simulink model "part_d_sim"  (R2019a)
settings: Solver=FixedStepAuto  StartTime=0.0  StopTime=10.0  FixedStep=0.01  RelTol=1e-3
undefined symbols (not defined in the file): A, B, C, D, R, sigbuilder_block
settings Model: Creator=Ranjani Kripashankar  LastModifiedBy=reema
settings DataIOCC: ReturnWorkspaceOutputs=off
settings DebuggingCC: ArithmeticOperatorsInVariantConditions=warning
settings SFSimCC: SimUseLocalCustomCode=off
settings RTWCC: RTWUseLocalCustomCode=off

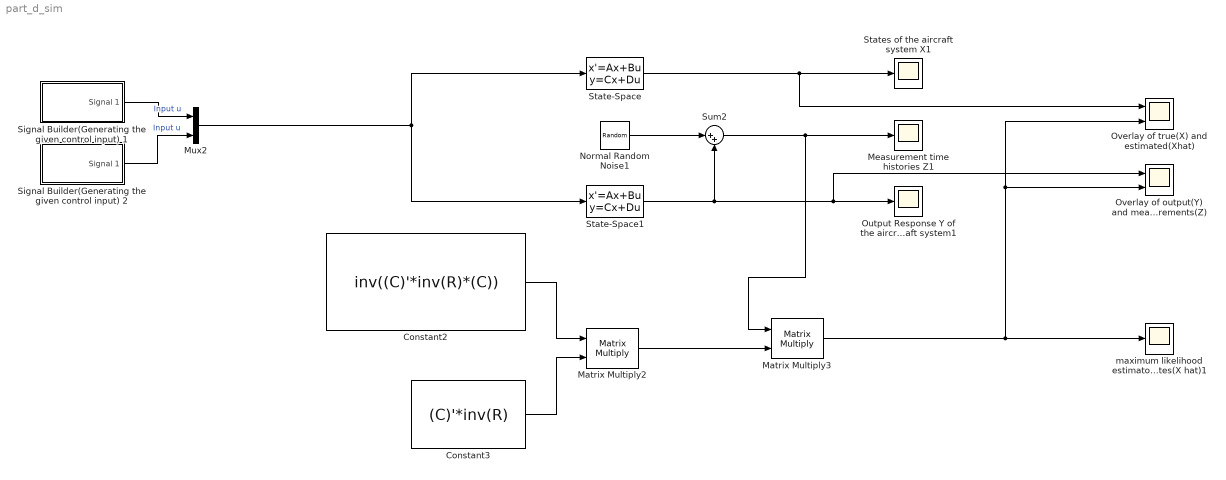
== system part_d_sim ==
  Constant2 : Constant  Value=inv((C)'*inv(R)*(C))
  Constant3 : Constant  Value=(C)'*inv(R)
  Matrix Multiply2 : Product  Multiplication=Matrix(*)
  Matrix Multiply3 : Product  Multiplication=Matrix(*)
  Measurement time histories Z1 : Scope
  Mux2 : Mux  Inputs=2
  Normal Random Noise1 : RandomNumber  Variance="[0.01  0.01  0.01  0.08]"  Seed=[1 2 3 4]  SampleTime=0.01
  Output Response Y of the aircraft system1 : Scope
  Overlay of output(Y) and measurements(Z) : Scope  NumInputPorts=2
  Overlay of true(X) and estimated(Xhat) : Scope  NumInputPorts=2
  Signal Builder(Generating the given control input) 1 : Subsystem  Tag=STV Subsys  LoadFcn=sigbuilder_block('load');  StartFcn=sigbuilder_block('start');  StopFcn=sigbuilder_block('stop');  ClipboardFcn=sigbuilder_block('clipboard');  mask(Sigbuilder block){tuvar=[0:10]}
      mask help: Simulink:masks:SigbuilderBlock_MD
      mask init:
      | if ~strcmp(get_param(bdroot(gcbh),'SimulationStatus'),'stopped') tuvar = sigbuilder_block('maskInit'); end
      settings: CopyFcn=sigbuilder_block('copy');  DeleteFcn=sigbuilder_block('delete');  ModelCloseFcn=sigbuilder_block('modelClose');  PreSaveFcn=sigbuilder_block('preSave');  PauseFcn=sigbuilder_block('pause');  ContinueFcn=sigbuilder_block('continue');  NameChangeFcn=sigbuilder_block('namechange');  OpenFcn=sigbuilder_block('open',[6 30 1012.5 447.75 ]);  CloseFcn=sigbuilder_block('close');
      mask Display: plot(0, 0, 100, 100,[2, 2, 32, 32, 2], [68, 8, 8, 68, 68],[32, 2], [38, 38], [32, 19, 2],[53, 60, 44], [32, 17, 17, 2],[16, 16, 31, 31]);txt = getActiveGroup(gcbh);text(2, 100, txt,'verticalAlignment', 'top');
  Signal Builder(Generating the given control input) 2 : Subsystem  Tag=STV Subsys  LoadFcn=sigbuilder_block('load');  StartFcn=sigbuilder_block('start');  StopFcn=sigbuilder_block('stop');  ClipboardFcn=sigbuilder_block('clipboard');  mask(Sigbuilder block){tuvar=[0:10]}
      mask help: Simulink:masks:SigbuilderBlock_MD
      mask init:
      | if ~strcmp(get_param(bdroot(gcbh),'SimulationStatus'),'stopped') tuvar = sigbuilder_block('maskInit'); end
      settings: CopyFcn=sigbuilder_block('copy');  DeleteFcn=sigbuilder_block('delete');  ModelCloseFcn=sigbuilder_block('modelClose');  PreSaveFcn=sigbuilder_block('preSave');  PauseFcn=sigbuilder_block('pause');  ContinueFcn=sigbuilder_block('continue');  NameChangeFcn=sigbuilder_block('namechange');  OpenFcn=sigbuilder_block('open',[6 30 1012.5 447.75 ]);  CloseFcn=sigbuilder_block('close');
      mask Display: plot(0, 0, 100, 100,[2, 2, 32, 32, 2], [68, 8, 8, 68, 68],[32, 2], [38, 38], [32, 19, 2],[53, 60, 44], [32, 17, 17, 2],[16, 16, 31, 31]);txt = getActiveGroup(gcbh);text(2, 100, txt,'verticalAlignment', 'top');
  State-Space : StateSpace  A=A  B=B  C=C  D=D  InitialCondition=0
  State-Space1 : StateSpace  A=A  B=B  C=C  D=D  InitialCondition=0
  States of the aircraft system X1 : Scope
  Sum2 : Sum  Inputs=|++
  maximum likelihood estimator estimated states(X hat)1 : Scope
  wires:
  Signal Builder(Generating the given control input) 2/1(Signal 1) -> Mux2/2  "Input u"
  Mux2/1 -> State-Space1/1, State-Space/1
  Sum2/1 -> Matrix Multiply3/1, Measurement time histories Z1/1
  Signal Builder(Generating the given control input) 1/1(Signal 1) -> Mux2/1  "Input u"
  Normal Random Noise1/1 -> Sum2/1
  State-Space/1 -> Overlay of true(X) and estimated(Xhat)/1, States of the aircraft system X1/1
  State-Space1/1 -> Overlay of output(Y) and measurements(Z)/1, Output Response Y of the aircraft system1/1, Sum2/2
  Matrix Multiply3/1 -> Overlay of output(Y) and measurements(Z)/2, Overlay of true(X) and estimated(Xhat)/2, maximum likelihood estimator estimated states(X hat)1/1
  Constant3/1 -> Matrix Multiply2/2
  Constant2/1 -> Matrix Multiply2/1
  Matrix Multiply2/1 -> Matrix Multiply3/2

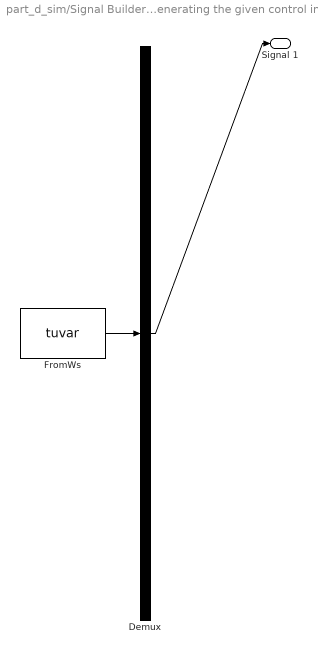
== system part_d_sim/Signal Builder(Generating the given control input) 1 ==
  Demux : Demux  Tag=STV Demux  Outputs=1
  FromWs : FromWorkspace  Tag=STV FromWs  VariableName=tuvar  SampleTime=0
      SigBuilderData=|
      | common.afterFinalStr = 'Extrapolate'
      | common.sampleTime = 0
      | dataSet.timeRange = [0 10]
      | dataSet.name = 'Group 1'
      | sbobj.Groups.Name = 'Group 1'
      | sbobj.Groups.Signals.Name = 'Signal 1'
      | sbobj.Groups.Signals.XData = [0 1 1 2 2 3 3 4 5 6 7 8 9 10]
      | sbobj.Groups.Signals.YData = [0 0 50 50 -50 -50 0 0 0 0 0 0 0 0]
  Signal 1 : Outport  Tag=STV Outport
  wires:
  FromWs/1 -> Demux/1
  Demux/1 -> Signal 1/1

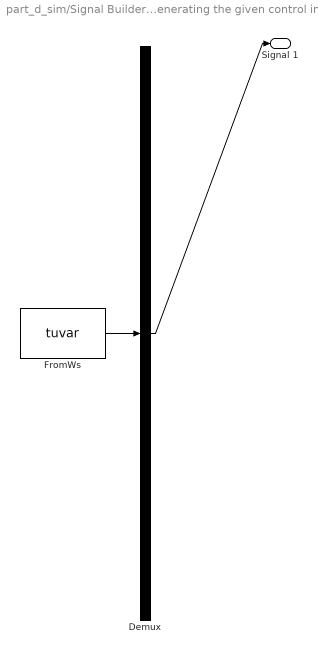
== system part_d_sim/Signal Builder(Generating the given control input) 2 ==
  Demux : Demux  Tag=STV Demux  Outputs=1
  FromWs : FromWorkspace  Tag=STV FromWs  VariableName=tuvar  SampleTime=0
      SigBuilderData=|
      | common.afterFinalStr = 'Extrapolate'
      | common.sampleTime = 0
      | dataSet.timeRange = [0 10]
      | dataSet.name = 'Group 1'
      | sbobj.Groups.Name = 'Group 1'
      | sbobj.Groups.Signals.Name = 'Signal 1'
      | sbobj.Groups.Signals.XData = [0 1 1 2 2 3 3 4 5 6 7 8 9 10]
      | sbobj.Groups.Signals.YData = [0 0 50 50 -50 -50 0 0 0 0 0 0 0 0]
  Signal 1 : Outport  Tag=STV Outport
  wires:
  FromWs/1 -> Demux/1
  Demux/1 -> Signal 1/1
